simulink model "BEV_maxSpeed"  (R2023a)
settings: Solver=FixedStepAuto  StartTime=0.0  StopTime=1000  FixedStep=1  RelTol=1e-3
undefined symbols (not defined in the file): acceleration_threshold, attributes, battery_GD, config_gearbox, config_Inverter, config_motor, config_vehicle, efficiency_vector, efficiency_vector2, GB, gearbox_map, k_FW, lossData, lossData2, max_torque_map, max_torque_map2, speed_vector, speed_vector2
libraries: spsParallelRLCBranchLib x20, spsControlledCurrentSourceLib x8, spsVoltageMeasurementLib x8, simulink x4, spsDCVoltageSourceLib x4, spspowerguiLib x4, eePmsmCurrentReferenceGen x2
(part 1 of 2)
settings Model: PauseTimes=35  Creator=maximilian.tschochne  LastModifiedBy=polashehata
settings OptimizationCC: ReuseModelBlockBuffer=off
settings DebuggingCC: MergeDetectMultiDrivingBlocksExec=none
settings ModelReferenceCC: PropagateSignalLabelsOutOfModel=off
settings RTWCC: GenCodeOnly=on  GenerateReport=on  BuildConfiguration=Faster Runs  CheckMdlBeforeBuild=Warning
settings GRTTargetCC: TargetLangStandard=C89/C90 (ANSI)  CodeInterfacePackaging=Reusable function  GenerateAllocFcn=on

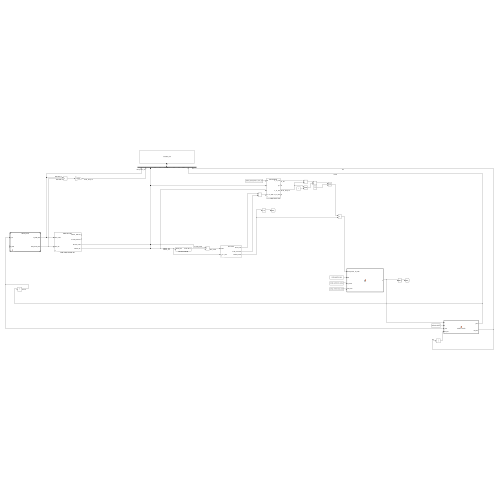
[thumbnail: Simulink's stored preview of the top-level diagram]
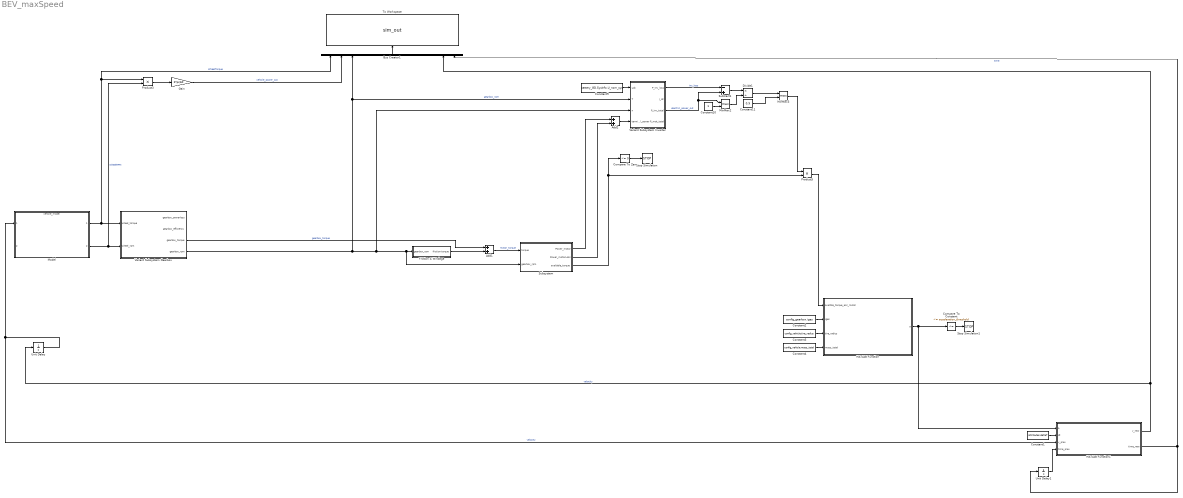
== system BEV_maxSpeed ==
  Add1 : Sum
  Add2 : Sum
  Bus Creator1 : BusCreator  Inputs=12
  Compare To Constant : simulink/Logic and Bit Operations/Compare To Constant  relop=<=  const=acceleration_threshold  OutDataTypeStr=boolean
  Compare To Zero : simulink/Logic and Bit Operations/Compare To Zero  relop=<=  OutDataTypeStr=boolean
  Constant1 : Constant  Value=attributes.deltaT
  Constant10 : Constant
  Constant11 : Constant  Value=0.9
  Constant2 : Constant  Value=config_gearbox.iges
  Constant3 : Constant  Value=config_vehicle.tire_radius
  Constant4 : Constant  Value=config_vehicle.mass_total
  Constant9 : Constant  Value=battery_GD.SysInfo.U_nom_sys
  Divide1 : Product  Inputs=*/
  Friction & Windage : Subsystem
  Gain : Gain  Gain=2*pi/60
  MATLAB Function : MATLAB Function  TreatAsAtomicUnit=on
  MATLAB Function1 : MATLAB Function  TreatAsAtomicUnit=on
  MinMax2 : MinMax  Function=max  Inputs=2
  MinMax3 : MinMax  Function=max  Inputs=2
  Model : ModelReference  ModelNameDialog=vehicle_model.slx  SimulationMode=Normal  ModelReferenceVersion=4.1
  Product3 : Product
  Product5 : Product
  Stop Simulation : Stop
  Stop Simulation1 : Stop
  Subsystem : Subsystem  Variant=on  VariantControl=Subsystem
  Subtract1 : Sum  Inputs=-+
  To Workspace : ToWorkspace  VariableName=sim_out  SaveFormat=Timeseries  SampleTime=-1
  Unit Delay : UnitDelay  SampleTime=-1  HasFrameUpgradeWarning=on
  Unit Delay1 : UnitDelay  SampleTime=-1  HasFrameUpgradeWarning=on
  Variant Subsystem Gearbox : Subsystem  Variant=on
  Variant Subsystem Inverter : Subsystem  Variant=on
  wires:
  Bus Creator1/1 -> To Workspace/1
  Gain/1 -> Bus Creator1/2  "vehicle_power_out"
  Model/2 -> Product3/2, Variant Subsystem Gearbox/2(wheel_rpm)  "WheelRPM"
  Model/1 -> Bus Creator1/1, Product3/1, Variant Subsystem Gearbox/1(wheel_torque)  "WheelTorque"
  Product3/1 -> Gain/1
  Constant1/1 -> MATLAB Function1/2(dt)
  MATLAB Function/1(a) -> MATLAB Function1/1(a), Compare To Constant/1
  MATLAB Function1/1(v_new) -> Unit Delay/1, Bus Creator1/11  "velocity"
  MATLAB Function1/2(time_new) -> Bus Creator1/12, Unit Delay1/1  "time"
  Add1/1 -> Subsystem/1(torque)  "motor_torque"
  Variant Subsystem Gearbox/3(gearbox_torque) -> Add1/1  "gearbox_torque"
  Variant Subsystem Gearbox/4(gearbox_rpm) -> Subsystem/2(gearbox_rpm), Friction & Windage/1(gearbox_rpm), Variant Subsystem Inverter/3(n), Bus Creator1/3, Variant Subsystem Inverter/2(T)  "gearbox_rpm"
  Friction & Windage/1(friction torque) -> Add1/2
  Constant2/1 -> MATLAB Function/2(iges)
  Constant3/1 -> MATLAB Function/3(tire_radius)
  Constant4/1 -> MATLAB Function/4(mass_total)
  Unit Delay1/1 -> MATLAB Function1/4(time_prev)
  Unit Delay/1 -> Model/1, MATLAB Function1/3(v_prev)  "velocity"
  Compare To Zero/1 -> Stop Simulation/1
  Compare To Constant/1 -> Stop Simulation1/1
  Constant9/1 -> Variant Subsystem Inverter/1(udc)
  Add2/1 -> Variant Subsystem Inverter/4(terminal_power)
  Variant Subsystem Inverter/3(P_inv_total) -> Subtract1/2, MinMax2/1  "electric_power_out"
  Variant Subsystem Inverter/1(P_inv_loss) -> Subtract1/1  "inv_loss"
  Subtract1/1 -> Divide1/1
  Divide1/1 -> MinMax3/1
  Product5/1 -> MATLAB Function/1(availble_torque_acc_motor)
  Constant10/1 -> MinMax2/2
  MinMax2/1 -> Divide1/2
  Constant11/1 -> MinMax3/2
  MinMax3/1 -> Product5/1
  Subsystem/1(Power_motor) -> Add2/1
  Subsystem/2(Power_motorLoss) -> Add2/2
  Subsystem/3(available_torque) -> Product5/2, Compare To Zero/1

== system BEV_maxSpeed/Friction & Windage ==
  note: Gleichung für mechanische Verlustleistung:
      | P_FW = k_FW * n^2.5
  gearbox_rpm : Inport
  Constant : Constant  Value=2.5
  Constant1 : Constant  Value=0
  Constant5 : Constant  Value=k_FW
  Gain : Gain  Gain=2*pi/60
  In2 : InportShadow
  Power : Math  Operator=pow
  Product : Product
  Product2 : Product  Inputs=*/
  Switch : Switch  Criteria=u2 > Threshold  SaturateOnIntegerOverflow=off  InputSameDT=off
  friction torque : Outport
  wires:
  gearbox_rpm/1 -> Power/1  "n_gearbox"
  Constant/1 -> Power/2  "exponent"
  Power/1 -> Product/1
  Constant5/1 -> Product/2
  Product/1 -> Product2/1  "mech powerloss"
  Product2/1 -> Switch/1  "torque"
  In2/1 -> Gain/1  "n_gearbox"
  Gain/1 -> Product2/2, Switch/2
  Switch/1 -> friction torque/1
  Constant1/1 -> Switch/3

== system BEV_maxSpeed/Subsystem ==
  torque : Inport
  gearbox_rpm : Inport  Port=2
  One Motor : Subsystem  VariantControl="Motor_Mode == \"LookupOneMotor\""
  Two motors : Subsystem  VariantControl="Motor_Mode == \"Lookup\""
  Power_motor : Outport
  Power_motorLoss : Outport  Port=2
  available_torque : Outport  Port=3

== system BEV_maxSpeed/Variant Subsystem Gearbox ==
  note: 1) Add Subsystem or Model blocks as valid variant choices.
      | 2) You cannot connect blocks at this level. At simulation, connectivity is automatically
      | determined, based on the active variant and port name matching.
  wheel_torque : Inport
  wheel_rpm : Inport  Port=2
  Gearbox Analytic : Subsystem  VariantControl="GB_Mode == \"Analytic\""
  Gearbox Const : Subsystem  VariantControl="GB_Mode == \"Const\""
  Gearbox Lookup-Table : Subsystem  VariantControl="GB_Mode == \"Lookup\""
  Gearbox Simple : Subsystem  VariantControl="GB_Mode == \"Simple\""
  gearbox_powerloss : Outport
  gearbox_efficiency : Outport  Port=2
  gearbox_torque : Outport  Port=3
  gearbox_rpm : Outport  Port=4

== system BEV_maxSpeed/Variant Subsystem Inverter ==
  note: 1) Add Subsystem or Model blocks as valid variant choices.
      | 2) You cannot connect blocks at this level. At simulation, connectivity is automatically
      | determined, based on the active variant and port name matching.
  udc : Inport
  T : Inport  Port=2
  n : Inport  Port=3
  terminal_power : Inport  Port=4
  Inverter Analytic : Subsystem  VariantControl="Inverter_Mode == \"Analytic\""
  Inverter Simple : Subsystem  VariantControl="Inverter_Mode == \"Simple\""
  P_inv_loss : Outport
  I_dc : Outport  Port=2
  P_inv_total : Outport  Port=3
  P_mot_total : Outport  Port=4

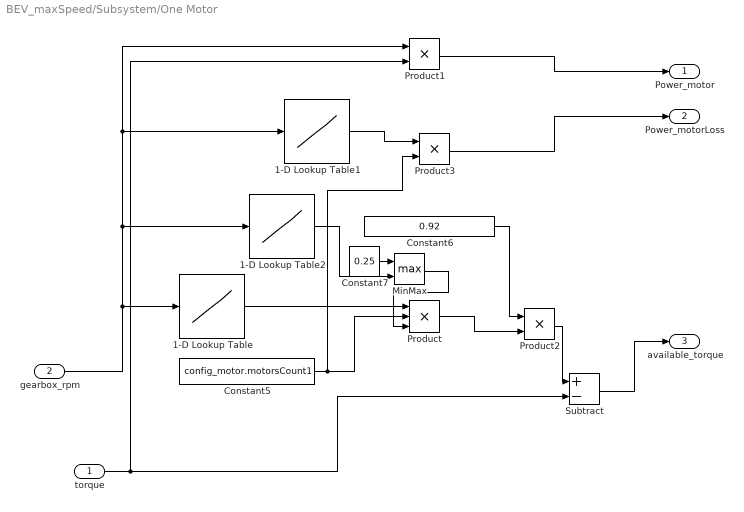
== system BEV_maxSpeed/Subsystem/One Motor ==
  torque : Inport
  gearbox_rpm : Inport  Port=2
  1-D Lookup Table : Lookup_n-D  NumberOfTableDimensions=1  BreakpointsForDimension1=speed_vector  Table=max_torque_map  InternalRulePriority=Speed  RndMeth=Simplest
  1-D Lookup Table1 : Lookup_n-D  NumberOfTableDimensions=1  BreakpointsForDimension1=speed_vector  Table=lossData  InternalRulePriority=Speed  RndMeth=Simplest
  1-D Lookup Table2 : Lookup_n-D  NumberOfTableDimensions=1  BreakpointsForDimension1=speed_vector  Table=efficiency_vector  InternalRulePriority=Speed  RndMeth=Simplest
  Constant5 : Constant  Value=config_motor.motorsCount1
  Constant6 : Constant  Value=0.92
  Constant7 : Constant  Value=0.25
  MinMax : MinMax  Function=max  Inputs=2
  Product : Product  Inputs=3
  Product1 : Product
  Product2 : Product
  Product3 : Product
  Subtract : Sum  Inputs=+-
  Power_motor : Outport
  Power_motorLoss : Outport  Port=2
  available_torque : Outport  Port=3
  wires:
  Product2/1 -> Subtract/1
  Subtract/1 -> available_torque/1
  1-D Lookup Table2/1 -> MinMax/2
  Constant5/1 -> Product/2, Product3/2
  Constant7/1 -> MinMax/1
  MinMax/1 -> Product/3
  1-D Lookup Table/1 -> Product/1
  Constant6/1 -> Product2/1
  Product/1 -> Product2/2
  gearbox_rpm/1 -> 1-D Lookup Table/1, 1-D Lookup Table2/1, Product1/1, 1-D Lookup Table1/1
  torque/1 -> Product1/2, Subtract/2
  1-D Lookup Table1/1 -> Product3/1
  Product3/1 -> Power_motorLoss/1
  Product1/1 -> Power_motor/1

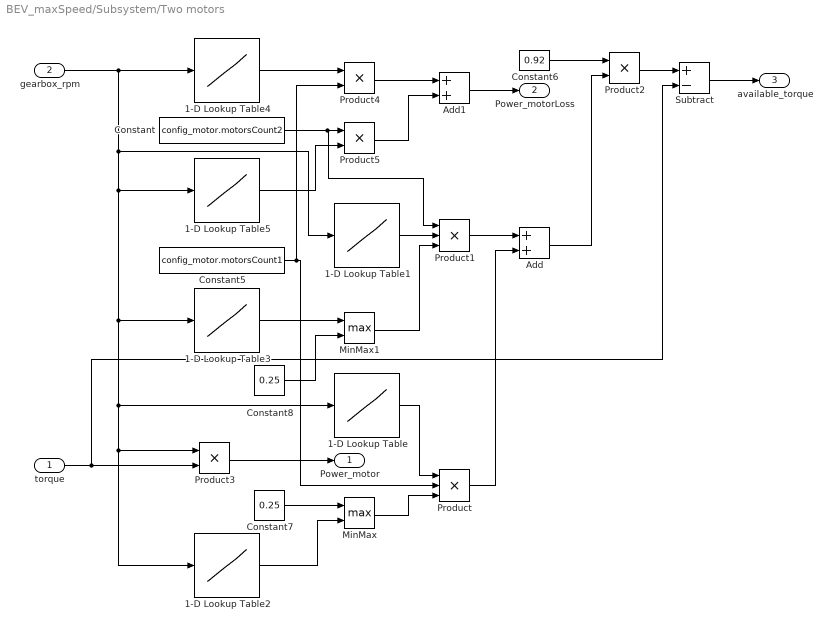
== system BEV_maxSpeed/Subsystem/Two motors ==
  torque : Inport
  gearbox_rpm : Inport  Port=2
  1-D Lookup Table : Lookup_n-D  NumberOfTableDimensions=1  BreakpointsForDimension1=speed_vector  Table=max_torque_map  InternalRulePriority=Speed  RndMeth=Simplest
  1-D Lookup Table1 : Lookup_n-D  NumberOfTableDimensions=1  BreakpointsForDimension1=speed_vector2  Table=max_torque_map2  InternalRulePriority=Speed  RndMeth=Simplest
  1-D Lookup Table2 : Lookup_n-D  NumberOfTableDimensions=1  BreakpointsForDimension1=speed_vector  Table=efficiency_vector  InternalRulePriority=Speed  RndMeth=Simplest
  1-D Lookup Table3 : Lookup_n-D  NumberOfTableDimensions=1  BreakpointsForDimension1=speed_vector2  Table=efficiency_vector2  InternalRulePriority=Speed  RndMeth=Simplest
  1-D Lookup Table4 : Lookup_n-D  NumberOfTableDimensions=1  BreakpointsForDimension1=speed_vector  Table=lossData  InternalRulePriority=Speed  RndMeth=Simplest
  1-D Lookup Table5 : Lookup_n-D  NumberOfTableDimensions=1  BreakpointsForDimension1=speed_vector2  Table=lossData2  InternalRulePriority=Speed  RndMeth=Simplest
  Add : Sum
  Add1 : Sum
  Constant : Constant  Value=config_motor.motorsCount2
  Constant5 : Constant  Value=config_motor.motorsCount1
  Constant6 : Constant  Value=0.92
  Constant7 : Constant  Value=0.25
  Constant8 : Constant  Value=0.25
  MinMax : MinMax  Function=max  Inputs=2
  MinMax1 : MinMax  Function=max  Inputs=2
  Product : Product  Inputs=3
  Product1 : Product  Inputs=3
  Product{2..5} (4 alike) : Product
  Subtract : Sum  Inputs=+-
  Power_motor : Outport
  Power_motorLoss : Outport  Port=2
  available_torque : Outport  Port=3
  wires:
  Subtract/1 -> available_torque/1
  1-D Lookup Table2/1 -> MinMax/2
  Product2/1 -> Subtract/1
  Add/1 -> Product2/2
  Constant6/1 -> Product2/1
  Product/1 -> Add/2
  Add1/1 -> Power_motorLoss/1
  1-D Lookup Table1/1 -> Product1/2
  Product5/1 -> Add1/2
  Constant7/1 -> MinMax/1
  MinMax/1 -> Product/3
  Product3/1 -> Power_motor/1
  Constant8/1 -> MinMax1/2
  1-D Lookup Table3/1 -> MinMax1/1
  Product1/1 -> Add/1
  Constant5/1 -> Product4/2, Product/2
  1-D Lookup Table4/1 -> Product4/1
  1-D Lookup Table/1 -> Product/1
  Constant/1 -> Product5/1, Product1/1
  torque/1 -> Product3/2, Subtract/2
  MinMax1/1 -> Product1/3
  Product4/1 -> Add1/1
  1-D Lookup Table5/1 -> Product5/2
  gearbox_rpm/1 -> Product3/1, 1-D Lookup Table2/1, 1-D Lookup Table/1, 1-D Lookup Table3/1, 1-D Lookup Table5/1, 1-D Lookup Table1/1, 1-D Lookup Table4/1

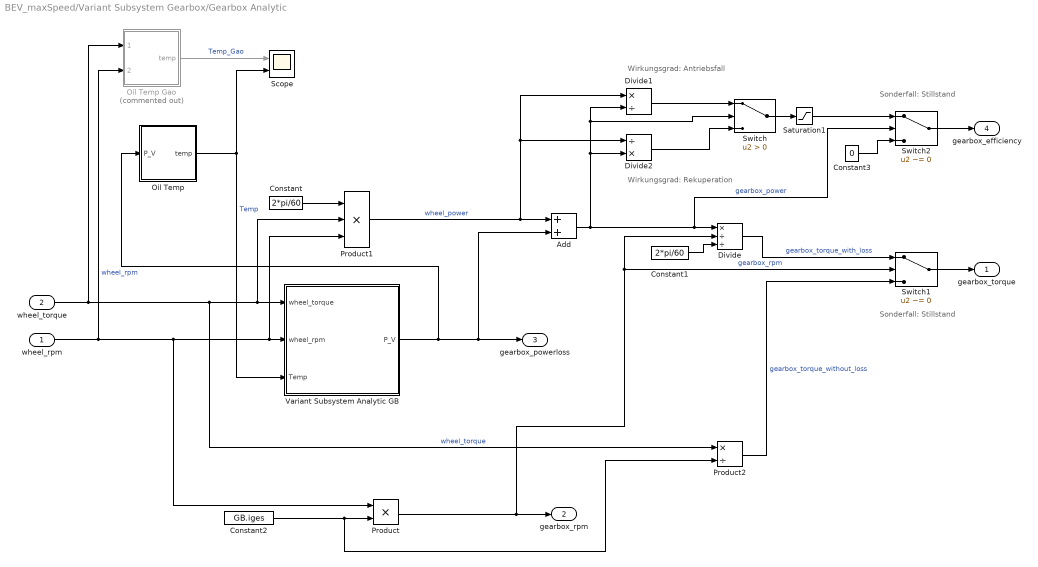
== system BEV_maxSpeed/Variant Subsystem Gearbox/Gearbox Analytic ==
  note: Wirkungsgrad:
      | Antriebsfall
  note: Sonderfall: Stillstand
  note: Sonderfall: Stillstand
  note: Wirkungsgrad:
      | Rekuperation
  wheel_rpm : Inport
  wheel_torque : Inport  Port=2
  Add : Sum
  Constant : Constant  Value=2*pi/60
  Constant1 : Constant  Value=2*pi/60
  Constant2 : Constant  Value=GB.iges
  Constant3 : Constant  Value=0
  Divide : Product  Inputs=*//
  Divide1 : Product  Inputs=*/
  Divide2 : Product  Inputs=/*
  Oil Temp : Subsystem
  Oil Temp Gao : Subsystem  Commented=on
  Product : Product
  Product1 : Product  Inputs=3
  Product2 : Product  Inputs=*/
  Saturation1 : Saturate  UpperLimit=inf  LowerLimit=0
  Scope : Scope  NumInputPorts=2
  Switch : Switch  Criteria=u2 > Threshold  SaturateOnIntegerOverflow=off  InputSameDT=off
  Switch1 : Switch  Criteria=u2 ~= 0  SaturateOnIntegerOverflow=off  InputSameDT=off
  Switch2 : Switch  Criteria=u2 ~= 0  SaturateOnIntegerOverflow=off  InputSameDT=off
  Variant Subsystem Analytic GB : Subsystem  Variant=on
  gearbox_torque : Outport
  gearbox_rpm : Outport  Port=2
  gearbox_powerloss : Outport  Port=3
  gearbox_efficiency : Outport  Port=4
  wires:
  wheel_torque/1 -> Variant Subsystem Analytic GB/1(wheel_torque), Product1/2, Product2/1, Oil Temp Gao/1(T_wheel)  "wheel_torque"
  wheel_rpm/1 -> Product/1, Variant Subsystem Analytic GB/2(wheel_rpm), Product1/3, Oil Temp Gao/2(rpm_wheel)  "wheel_rpm"
  Variant Subsystem Analytic GB/1(P_V) -> Oil Temp/1(P_V), Add/2, gearbox_powerloss/1
  Constant2/1 -> Product2/2, Product/2
  Product/1 -> Switch1/2, Divide/2, gearbox_rpm/1  "gearbox_rpm"
  Constant/1 -> Product1/1
  Product1/1 -> Divide2/1, Divide1/1, Add/1  "wheel_power"
  Add/1 -> Divide2/2, Switch/2, Divide1/2, Switch2/2, Divide/1  "gearbox_power"
  Constant1/1 -> Divide/3
  Divide/1 -> Switch1/1  "gearbox_torque_with_loss"
  Switch/1 -> Saturation1/1
  Divide2/1 -> Switch/3
  Switch1/1 -> gearbox_torque/1
  Product2/1 -> Switch1/3  "gearbox_torque_without_loss"
  Switch2/1 -> gearbox_efficiency/1
  Constant3/1 -> Switch2/3
  Divide1/1 -> Switch/1
  Oil Temp Gao/1(temp) -> Scope/1  "Temp_Gao"
  Oil Temp/1(temp) -> Scope/2, Variant Subsystem Analytic GB/3(Temp)  "Temp"
  Saturation1/1 -> Switch2/1

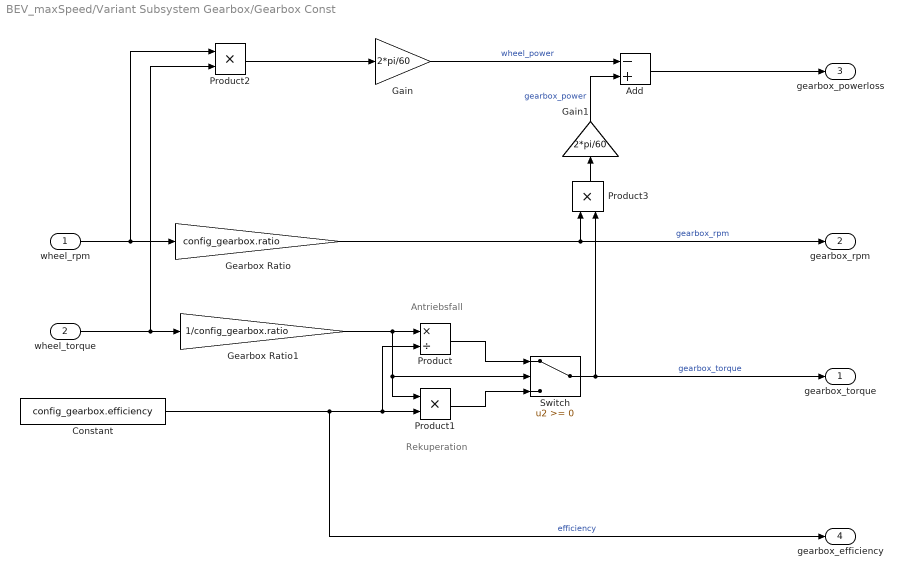
== system BEV_maxSpeed/Variant Subsystem Gearbox/Gearbox Const ==
  note: Rekuperation
  note: Antriebsfall
  wheel_rpm : Inport
  wheel_torque : Inport  Port=2
  Add : Sum  Inputs=-+
  Constant : Constant  Value=config_gearbox.efficiency
  Gain : Gain  Gain=2*pi/60
  Gain1 : Gain  Gain=2*pi/60
  Gearbox Ratio : Gain  Gain=config_gearbox.ratio
  Gearbox Ratio1 : Gain  Gain=1/config_gearbox.ratio
  Product : Product  Inputs=*/
  Product1 : Product  Inputs=**
  Product2 : Product
  Product3 : Product
  Switch : Switch  SaturateOnIntegerOverflow=off  InputSameDT=off
  gearbox_torque : Outport
  gearbox_rpm : Outport  Port=2
  gearbox_powerloss : Outport  Port=3
  gearbox_efficiency : Outport  Port=4
  wires:
  wheel_rpm/1 -> Product2/1, Gearbox Ratio/1
  Gearbox Ratio/1 -> gearbox_rpm/1, Product3/1  "gearbox_rpm"
  wheel_torque/1 -> Product2/2, Gearbox Ratio1/1
  Gearbox Ratio1/1 -> Product1/1, Switch/2, Product/1
  Constant/1 -> gearbox_efficiency/1, Product1/2, Product/2  "efficiency"
  Product/1 -> Switch/1
  Product1/1 -> Switch/3
  Switch/1 -> gearbox_torque/1, Product3/2  "gearbox_torque"
  Product2/1 -> Gain/1
  Add/1 -> gearbox_powerloss/1
  Product3/1 -> Gain1/1
  Gain/1 -> Add/1  "wheel_power"
  Gain1/1 -> Add/2  "gearbox_power"

== system BEV_maxSpeed/Variant Subsystem Gearbox/Gearbox Lookup-Table ==
  wheel_rpm : Inport
  wheel_torque : Inport  Port=2
  Oil Temp : Subsystem
  Oil Temp Gao : Subsystem  Commented=on
  Scope : Scope  Commented=on  NumInputPorts=2
  Variant Subsystem : Subsystem  Variant=on
  gearbox_torque : Outport
  gearbox_rpm : Outport  Port=2
  gearbox_powerloss : Outport  Port=3
  gearbox_efficiency : Outport  Port=4
  wires:
  Oil Temp Gao/1(temp) -> Scope/2
  wheel_torque/1 -> Oil Temp Gao/1(T_wheel), Variant Subsystem/1(wheel_torque)  "wheel_torque"
  wheel_rpm/1 -> Oil Temp Gao/2(rpm_wheel), Variant Subsystem/2(wheel_rpm)  "wheel_rpm"
  Variant Subsystem/4(gearbox_torque) -> gearbox_torque/1
  Variant Subsystem/1(loss_lockup) -> Oil Temp/1(P_V), gearbox_powerloss/1
  Variant Subsystem/3(gearbox_rpm) -> gearbox_rpm/1
  Variant Subsystem/2(gearbox_efficiency) -> gearbox_efficiency/1
  Oil Temp/1(temp) -> Scope/1, Variant Subsystem/3(Temp)

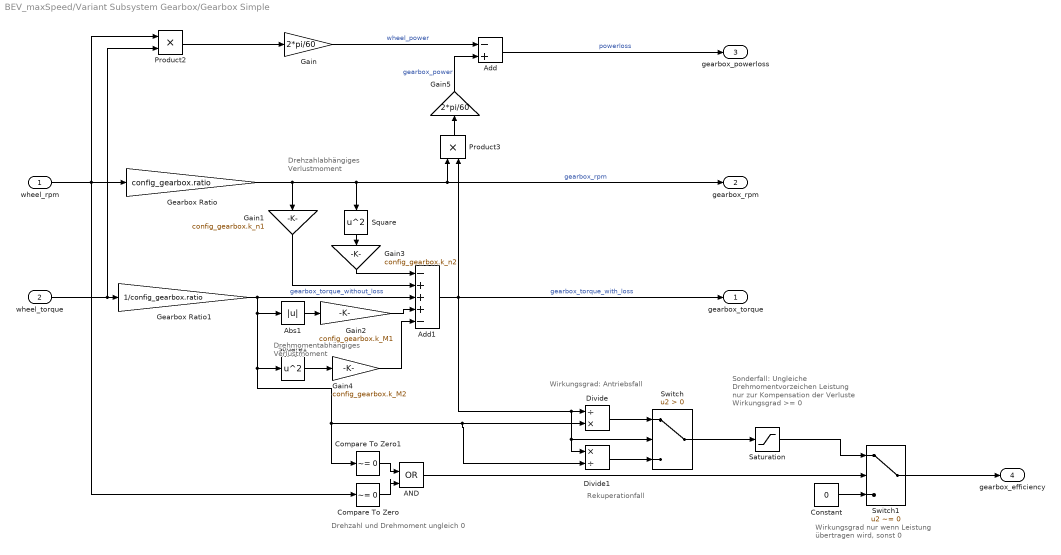
== system BEV_maxSpeed/Variant Subsystem Gearbox/Gearbox Simple ==
  note: Rekuperationfall
  note: Sonderfall: Ungleiche Drehmomentvorzeichen
      | Leistung nur zur Kompensation der Verluste
      | Wirkungsgrad >= 0
  note: Drehzahl und Drehmoment ungleich 0
  note: Drehmomentabhängiges
      | Verlustmoment
  note: Drehzahlabhängiges
      | Verlustmoment
  note: Wirkungsgrad nur wenn Leistung
      | übertragen wird, sonst 0
  note: Wirkungsgrad: Antriebsfall
  wheel_rpm : Inport
  wheel_torque : Inport  Port=2
  AND : Logic  Operator=OR  IconShape=distinctive  AllPortsSameDT=off  OutDataTypeStr=boolean
  Abs1 : Abs  SaturateOnIntegerOverflow=off
  Add : Sum  Inputs=-+
  Add1 : Sum  Inputs=-+++-
  Compare To Zero : simulink/Logic and Bit Operations/Compare To Zero  relop=~=  OutDataTypeStr=boolean
  Compare To Zero1 : simulink/Logic and Bit Operations/Compare To Zero  relop=~=  OutDataTypeStr=boolean
  Constant : Constant  Value=0
  Divide : Product  Inputs=/*
  Divide1 : Product  Inputs=*/
  Gain : Gain  Gain=2*pi/60
  Gain1 : Gain  Gain=config_gearbox.k_n1
  Gain2 : Gain  Gain=config_gearbox.k_M1
  Gain3 : Gain  Gain=config_gearbox.k_n2
  Gain4 : Gain  Gain=config_gearbox.k_M2
  Gain5 : Gain  Gain=2*pi/60
  Gearbox Ratio : Gain  Gain=config_gearbox.ratio
  Gearbox Ratio1 : Gain  Gain=1/config_gearbox.ratio
  Product2 : Product
  Product3 : Product
  Saturation : Saturate  UpperLimit=inf  LowerLimit=0
  Square : Math  Operator=square
  Square1 : Math  Operator=square
  Switch : Switch  Criteria=u2 > Threshold  SaturateOnIntegerOverflow=off  InputSameDT=off
  Switch1 : Switch  Criteria=u2 ~= 0  SaturateOnIntegerOverflow=off  InputSameDT=off
  gearbox_torque : Outport
  gearbox_rpm : Outport  Port=2
  gearbox_powerloss : Outport  Port=3
  gearbox_efficiency : Outport  Port=4
  wires:
  Product3/1 -> Gain5/1
  Add/1 -> gearbox_powerloss/1  "powerloss"
  Add1/1 -> Product3/2, gearbox_torque/1, Switch/2, Divide1/1, Divide/1  "gearbox_torque_with_loss"
  wheel_torque/1 -> Product2/2, Gearbox Ratio1/1
  Gearbox Ratio/1 -> Square/1, Product3/1, gearbox_rpm/1, Gain1/1  "gearbox_rpm"
  wheel_rpm/1 -> Compare To Zero/1, Gearbox Ratio/1, Product2/1
  Gearbox Ratio1/1 -> Abs1/1, Square1/1, Compare To Zero1/1, Divide1/2, Divide/2, Add1/3  "gearbox_torque_without_loss"
  Gain1/1 -> Add1/2
  Gain2/1 -> Add1/4
  Abs1/1 -> Gain2/1
  Divide/1 -> Switch/1
  Switch/1 -> Saturation/1
  Divide1/1 -> Switch/3
  Constant/1 -> Switch1/3
  Gain3/1 -> Add1/1
  Square/1 -> Gain3/1
  Switch1/1 -> gearbox_efficiency/1
  Square1/1 -> Gain4/1
  Gain4/1 -> Add1/5
  Compare To Zero1/1 -> AND/1
  Compare To Zero/1 -> AND/2
  AND/1 -> Switch1/2
  Product2/1 -> Gain/1
  Gain/1 -> Add/1  "wheel_power"
  Gain5/1 -> Add/2  "gearbox_power"
  Saturation/1 -> Switch1/1

== system BEV_maxSpeed/Variant Subsystem Inverter/Inverter Analytic ==
  udc : Inport
  T : Inport  Port=2
  n : Inport  Port=3
  terminal_power : Inport  Port=4
  Variant Subsystem : Subsystem  Variant=on
  P_inv_loss : Outport
  I_dc : Outport  Port=2
  P_inv_total : Outport  Port=3
  P_mot_total : Outport  Port=4
  wires:
  Variant Subsystem/4(P_mot_elec) -> P_mot_total/1
  Variant Subsystem/3(P_inv_total) -> P_inv_total/1
  Variant Subsystem/2(idc) -> I_dc/1
  Variant Subsystem/1(Conduction_and_Switching_loss) -> P_inv_loss/1
  T/1 -> Variant Subsystem/3(torque)
  n/1 -> Variant Subsystem/2(rpm)
  udc/1 -> Variant Subsystem/1(udc)
  terminal_power/1 -> Variant Subsystem/4(terminal_power)

== system BEV_maxSpeed/Variant Subsystem Inverter/Inverter Simple ==
  T : Inport
  n : Inport  Port=2
  udc : Inport  Port=3
  terminal_power : Inport  Port=4
  MATLAB Function : MATLAB Function  TreatAsAtomicUnit=on
  P_inv_loss : Outport
  I_dc : Outport  Port=2
  P_inv_total : Outport  Port=3
  P_mot_total : Outport  Port=4
  wires:
  T/1 -> MATLAB Function/1(T)
  n/1 -> MATLAB Function/2(n)
  udc/1 -> MATLAB Function/3(udc)
  terminal_power/1 -> MATLAB Function/4(P_Terminal)
  MATLAB Function/1(P_inv_loss) -> P_inv_loss/1
  MATLAB Function/2(I_dc) -> I_dc/1
  MATLAB Function/3(P_inv_total) -> P_inv_total/1
  MATLAB Function/4(P_mot_total) -> P_mot_total/1

== system BEV_maxSpeed/Variant Subsystem Gearbox/Gearbox Analytic/Oil Temp ==
  P_V : Inport
  IC : InitialCondition  Value=25
  MATLAB Function : MATLAB Function  TreatAsAtomicUnit=on
  Memory1 : Memory  InitialCondition=config_vehicle.ambient_temp - 273
  Memory2 : Memory  InitialCondition=config_vehicle.ambient_temp - 273
  Scope : Scope
  temp : Outport
  wires:
  MATLAB Function/1(T) -> IC/1  "GB_temp"
  Memory1/1 -> MATLAB Function/1(t)
  P_V/1 -> Memory2/1
  IC/1 -> Scope/1, Memory1/1, temp/1
  Memory2/1 -> MATLAB Function/2(P_V)

== system BEV_maxSpeed/Variant Subsystem Gearbox/Gearbox Analytic/Oil Temp Gao ==
  note: entspricht 2pi/60 * 1e-3
  T_wheel : Inport
  rpm_wheel : Inport  Port=2
  MATLAB Function : MATLAB Function  TreatAsAtomicUnit=on
  Memory1 : Memory  InitialCondition=config_vehicle.ambient_temp - 273
  Multiply5 : Gain  Gain=1/9550
  Product2 : Product
  Scope : Scope
  temp : Outport
  wires:
  Product2/1 -> Multiply5/1
  rpm_wheel/1 -> MATLAB Function/3(rpm), Product2/2
  T_wheel/1 -> Product2/1
  MATLAB Function/1(T) -> Scope/1, Memory1/1, temp/1
  Memory1/1 -> MATLAB Function/1(t)
  Multiply5/1 -> MATLAB Function/2(P)

== system BEV_maxSpeed/Variant Subsystem Gearbox/Gearbox Analytic/Variant Subsystem Analytic GB ==
  note: 1) Add Subsystem or Model blocks as valid variant choices.
      | 2) You cannot connect blocks at this level. At simulation, connectivity is automatically
      | determined, based on the active variant and port name matching.
  wheel_torque : Inport
  wheel_rpm : Inport  Port=2
  Temp : Inport  Port=3
  Einstufig_Achsparallel : Subsystem  VariantControl=GB_Stufen == 1
  Zweistufig_Achsparallel : Subsystem  VariantControl="GB_Stufen == 2 && GB_Topology == \"achsparallel\""
  Zweistufig_Koaxial : Subsystem  VariantControl="GB_Stufen == 2 && GB_Topology == \"koaxial\""
  P_V : Outport

== system BEV_maxSpeed/Variant Subsystem Gearbox/Gearbox Lookup-Table/Oil Temp ==
  P_V : Inport
  IC : InitialCondition  Value=25
  MATLAB Function : MATLAB Function  TreatAsAtomicUnit=on
  Memory1 : Memory  InitialCondition=config_vehicle.ambient_temp - 273
  Memory2 : Memory  InitialCondition=config_vehicle.ambient_temp - 273
  Scope : Scope
  temp : Outport
  wires:
  MATLAB Function/1(T) -> IC/1  "GB_temp"
  Memory1/1 -> MATLAB Function/1(t)
  P_V/1 -> Memory2/1
  IC/1 -> Scope/1, Memory1/1, temp/1
  Memory2/1 -> MATLAB Function/2(P_V)

== system BEV_maxSpeed/Variant Subsystem Gearbox/Gearbox Lookup-Table/Oil Temp Gao ==
  note: entspricht 2pi/60 * 1e-3
  T_wheel : Inport
  rpm_wheel : Inport  Port=2
  MATLAB Function : MATLAB Function  TreatAsAtomicUnit=on
  Memory1 : Memory  InitialCondition=config_vehicle.ambient_temp - 273
  Multiply5 : Gain  Gain=1/9550
  Product2 : Product
  Scope : Scope
  temp : Outport
  wires:
  Product2/1 -> Multiply5/1
  rpm_wheel/1 -> MATLAB Function/3(rpm), Product2/2
  T_wheel/1 -> Product2/1
  MATLAB Function/1(T) -> Scope/1, Memory1/1, temp/1
  Memory1/1 -> MATLAB Function/1(t)
  Multiply5/1 -> MATLAB Function/2(P)

== system BEV_maxSpeed/Variant Subsystem Gearbox/Gearbox Lookup-Table/Variant Subsystem ==
  note: 1) Add Subsystem or Model blocks as valid variant choices.
      | 2) You cannot connect blocks at this level. At simulation, connectivity is automatically
      | determined, based on the active variant and port name matching.
  wheel_torque : Inport
  wheel_rpm : Inport  Port=2
  Temp : Inport  Port=3
  ETA_map : Subsystem  VariantControl="gearbox_map.map_type == \"Eta\""
  LOSS_map : Subsystem  VariantControl="gearbox_map.map_type == \"Loss\""
  loss_lockup : Outport
  gearbox_efficiency : Outport  Port=2
  gearbox_rpm : Outport  Port=3
  gearbox_torque : Outport  Port=4

== system BEV_maxSpeed/Variant Subsystem Inverter/Inverter Analytic/Variant Subsystem ==
  note: 1) Add Subsystem or Model blocks as valid variant choices.
      | 2) You cannot connect blocks at this level. At simulation, connectivity is automatically
      | determined, based on the active variant and port name matching.
  udc : Inport
  rpm : Inport  Port=2
  torque : Inport  Port=3
  terminal_power : Inport  Port=4
  IM_Inverter_IGBT_Analytic : Subsystem  VariantControl=Mode_IM_IGBT
  IM_Inverter_SiC-MOSFET_Analytic : Subsystem  VariantControl=Mode_IM_MOSFET
  PMSM_Inverter_IBGT_Analytic : Subsystem  VariantControl=Mode_PSM_IGBT
  PMSM_Inverter_SiC-MOSFET_Analytic : Subsystem  VariantControl=Mode_PSM_MOSFET
  Conduction_and_Switching_loss : Outport
  idc : Outport  Port=2
  P_inv_total : Outport  Port=3
  P_mot_elec : Outport  Port=4

== system BEV_maxSpeed/Variant Subsystem Gearbox/Gearbox Analytic/Variant Subsystem Analytic GB/Einstufig_Achsparallel ==
  wheel_torque : Inport
  wheel_rpm : Inport  Port=2
  Temp : Inport  Port=3
  Add : Sum
  MATLAB Function : MATLAB Function  TreatAsAtomicUnit=on
  Ölpumpe : Subsystem
  P_V : Outport
  wires:
  wheel_rpm/1 -> Ölpumpe/1(nrad), MATLAB Function/2(nrad)
  MATLAB Function/1(P_V) -> Add/1
  wheel_torque/1 -> MATLAB Function/1(Mrad)
  Temp/1 -> MATLAB Function/3(Temp)
  Add/1 -> P_V/1
  Ölpumpe/1(power_oilpump) -> Add/2

== system BEV_maxSpeed/Variant Subsystem Gearbox/Gearbox Analytic/Variant Subsystem Analytic GB/Zweistufig_Achsparallel ==
  wheel_torque : Inport
  wheel_rpm : Inport  Port=2
  Temp : Inport  Port=3
  Add : Sum
  MATLAB Function : MATLAB Function  TreatAsAtomicUnit=on
  Ölpumpe : Subsystem
  P_V : Outport
  wires:
  wheel_rpm/1 -> Ölpumpe/1(nrad), MATLAB Function/2(nrad)
  MATLAB Function/1(P_V) -> Add/1
  wheel_torque/1 -> MATLAB Function/1(Mrad)
  Temp/1 -> MATLAB Function/3(Temp)
  Add/1 -> P_V/1
  Ölpumpe/1(power_oilpump) -> Add/2

== system BEV_maxSpeed/Variant Subsystem Gearbox/Gearbox Analytic/Variant Subsystem Analytic GB/Zweistufig_Koaxial ==
  wheel_torque : Inport
  wheel_rpm : Inport  Port=2
  Temp : Inport  Port=3
  Add : Sum
  MATLAB Function : MATLAB Function  TreatAsAtomicUnit=on
  Ölpumpe : Subsystem
  P_V : Outport
  wires:
  Temp/1 -> MATLAB Function/3(Temp)
  wheel_torque/1 -> MATLAB Function/1(Mrad)
  MATLAB Function/1(P_V) -> Add/1
  wheel_rpm/1 -> Ölpumpe/1(nrad), MATLAB Function/2(nrad)
  Add/1 -> P_V/1
  Ölpumpe/1(power_oilpump) -> Add/2

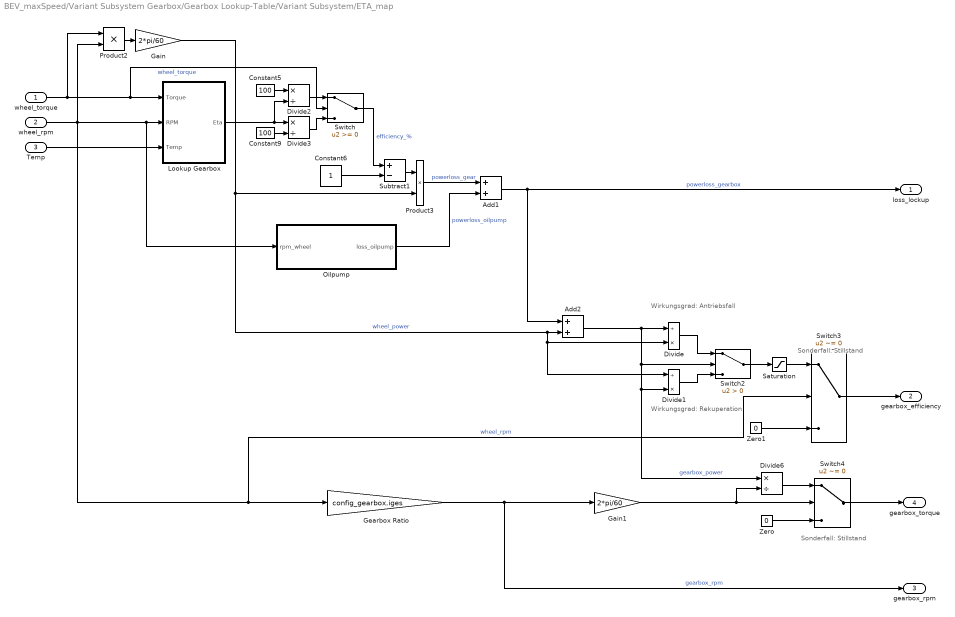
== system BEV_maxSpeed/Variant Subsystem Gearbox/Gearbox Lookup-Table/Variant Subsystem/ETA_map ==
  note: Sonderfall: Stillstand
  note: Sonderfall: Stillstand
  note: Wirkungsgrad:
      | Antriebsfall
  note: Wirkungsgrad:
      | Rekuperation
  wheel_torque : Inport
  wheel_rpm : Inport  Port=2
  Temp : Inport  Port=3
  Add1 : Sum
  Add2 : Sum
  Constant5 : Constant  Value=100
  Constant6 : Constant
  Constant9 : Constant  Value=100
  Divide : Product  Inputs=/*
  Divide1 : Product  Inputs=/*
  Divide2 : Product  Inputs=*/
  Divide3 : Product  Inputs=*/
  Divide6 : Product  Inputs=*/
  Gain : Gain  Gain=2*pi/60
  Gain1 : Gain  Gain=2*pi/60
  Gearbox Ratio : Gain  Gain=config_gearbox.iges
  Lookup Gearbox : Subsystem  Variant=on
  Oilpump : Subsystem
  Product2 : Product  Inputs=**
  Product3 : Product  Inputs=**
  Saturation : Saturate  UpperLimit=inf  LowerLimit=0
  Subtract1 : Sum  Inputs=+-
  Switch : Switch  SaturateOnIntegerOverflow=off  InputSameDT=off
  Switch2 : Switch  Criteria=u2 > Threshold  SaturateOnIntegerOverflow=off  InputSameDT=off
  Switch3 : Switch  Criteria=u2 ~= 0  SaturateOnIntegerOverflow=off  InputSameDT=off
  Switch4 : Switch  Criteria=u2 ~= 0  SaturateOnIntegerOverflow=off  InputSameDT=off
  Zero : Constant  Value=0  OutDataTypeStr=Inherit: Inherit via back propagation
  Zero1 : Constant  Value=0  OutDataTypeStr=Inherit: Inherit via back propagation
  loss_lockup : Outport
  gearbox_efficiency : Outport  Port=2
  gearbox_rpm : Outport  Port=3
  gearbox_torque : Outport  Port=4
  wires:
  wheel_torque/1 -> Lookup Gearbox/1(Torque), Switch/2, Product2/1  "wheel_torque"
  Divide1/1 -> Switch2/3
  Product2/1 -> Gain/1
  wheel_rpm/1 -> Switch3/2, Gearbox Ratio/1, Product2/2, Oilpump/1(rpm_wheel), Lookup Gearbox/2(RPM)  "wheel_rpm"
  Constant6/1 -> Subtract1/2
  Subtract1/1 -> Product3/1
  Switch/1 -> Subtract1/1  "efficiency_%"
  Product3/1 -> Add1/1  "powerloss_gear"
  Zero1/1 -> Switch3/3
  Switch2/1 -> Saturation/1
  Divide2/1 -> Switch/1
  Zero/1 -> Switch4/3
  Switch4/1 -> gearbox_torque/1
  Switch3/1 -> gearbox_efficiency/1
  Divide6/1 -> Switch4/1
  Gearbox Ratio/1 -> Gain1/1, gearbox_rpm/1  "gearbox_rpm"
  Divide3/1 -> Switch/3
  Add2/1 -> Switch2/2, Divide6/1, Divide1/2, Divide/1  "gearbox_power"
  Gain1/1 -> Switch4/2, Divide6/2
  Temp/1 -> Lookup Gearbox/3(Temp)
  Gain/1 -> Product3/2, Divide1/1, Divide/2, Add2/2  "wheel_power"
  Add1/1 -> Add2/1, loss_lockup/1  "powerloss_gearbox"
  Constant9/1 -> Divide3/2
  Oilpump/1(loss_oilpump) -> Add1/2  "powerloss_oilpump"
  Lookup Gearbox/1(Eta) -> Divide2/2, Divide3/1
  Divide/1 -> Switch2/1
  Constant5/1 -> Divide2/1
  Saturation/1 -> Switch3/1

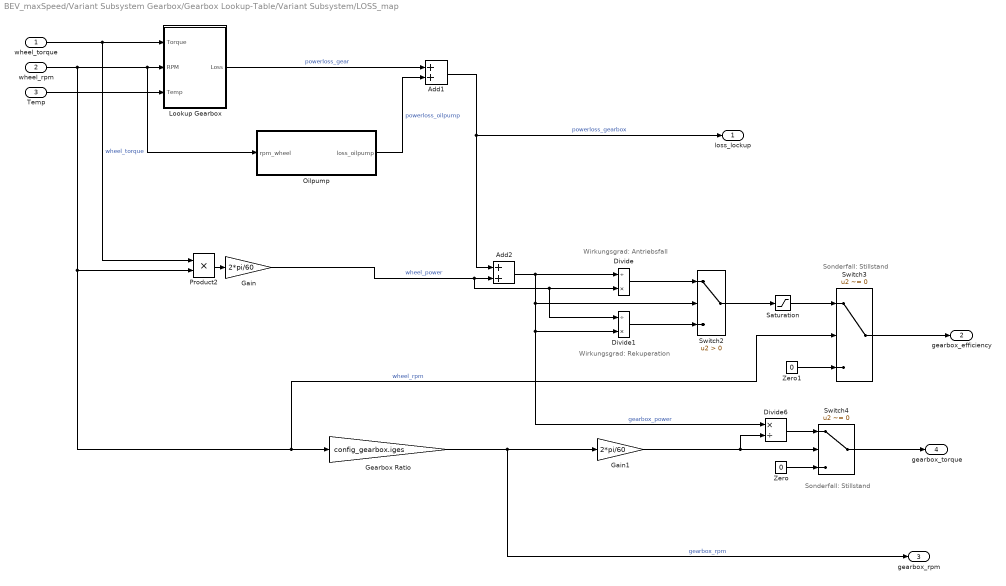
== system BEV_maxSpeed/Variant Subsystem Gearbox/Gearbox Lookup-Table/Variant Subsystem/LOSS_map ==
  note: Sonderfall: Stillstand
  note: Wirkungsgrad: Antriebsfall
  note: Wirkungsgrad: Rekuperation
  note: Sonderfall: Stillstand
  wheel_torque : Inport
  wheel_rpm : Inport  Port=2
  Temp : Inport  Port=3
  Add1 : Sum
  Add2 : Sum
  Divide : Product  Inputs=/*
  Divide1 : Product  Inputs=/*
  Divide6 : Product  Inputs=*/
  Gain : Gain  Gain=2*pi/60
  Gain1 : Gain  Gain=2*pi/60
  Gearbox Ratio : Gain  Gain=config_gearbox.iges
  Lookup Gearbox : Subsystem  Variant=on
  Oilpump : Subsystem
  Product2 : Product  Inputs=**
  Saturation : Saturate  UpperLimit=inf  LowerLimit=0
  Switch2 : Switch  Criteria=u2 > Threshold  SaturateOnIntegerOverflow=off  InputSameDT=off
  Switch3 : Switch  Criteria=u2 ~= 0  SaturateOnIntegerOverflow=off  InputSameDT=off
  Switch4 : Switch  Criteria=u2 ~= 0  SaturateOnIntegerOverflow=off  InputSameDT=off
  Zero : Constant  Value=0  OutDataTypeStr=Inherit: Inherit via back propagation
  Zero1 : Constant  Value=0  OutDataTypeStr=Inherit: Inherit via back propagation
  loss_lockup : Outport
  gearbox_efficiency : Outport  Port=2
  gearbox_rpm : Outport  Port=3
  gearbox_torque : Outport  Port=4
  wires:
  Gain/1 -> Divide1/1, Divide/2, Add2/2  "wheel_power"
  wheel_torque/1 -> Lookup Gearbox/1(Torque), Product2/1  "wheel_torque"
  Lookup Gearbox/1(Loss) -> Add1/1  "powerloss_gear"
  Product2/1 -> Gain/1
  Switch4/1 -> gearbox_torque/1
  Switch3/1 -> gearbox_efficiency/1
  Gearbox Ratio/1 -> gearbox_rpm/1, Gain1/1  "gearbox_rpm"
  Switch2/1 -> Saturation/1
  Divide/1 -> Switch2/1
  Add2/1 -> Divide/1, Switch2/2, Divide1/2, Divide6/1  "gearbox_power"
  Zero/1 -> Switch4/3
  Divide6/1 -> Switch4/1
  Divide1/1 -> Switch2/3
  Oilpump/1(loss_oilpump) -> Add1/2  "powerloss_oilpump"
  Add1/1 -> loss_lockup/1, Add2/1  "powerloss_gearbox"
  Temp/1 -> Lookup Gearbox/3(Temp)
  Gain1/1 -> Switch4/2, Divide6/2
  wheel_rpm/1 -> Switch3/2, Gearbox Ratio/1, Product2/2, Lookup Gearbox/2(RPM), Oilpump/1(rpm_wheel)  "wheel_rpm"
  Zero1/1 -> Switch3/3
  Saturation/1 -> Switch3/1

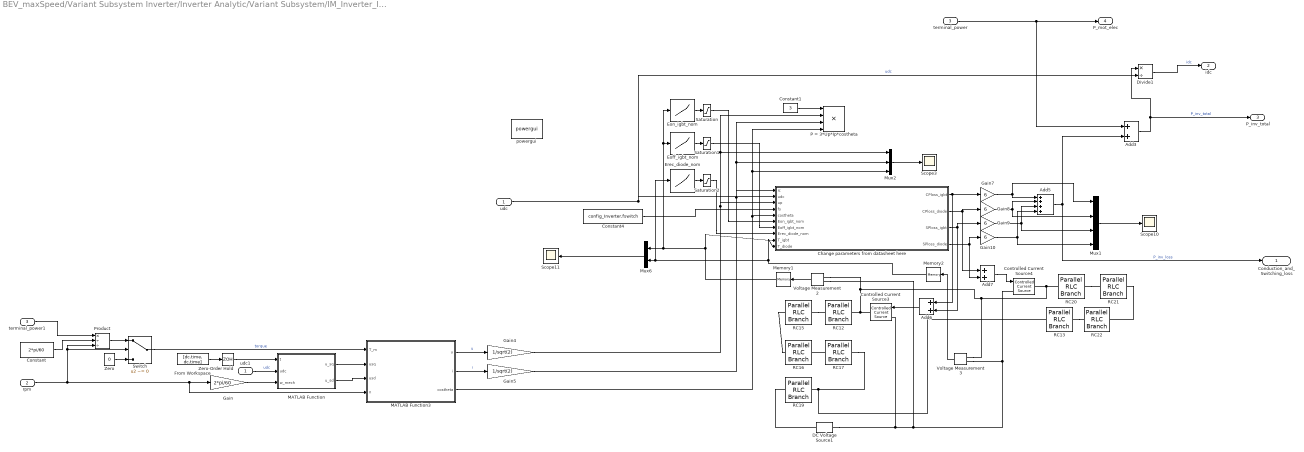
== system BEV_maxSpeed/Variant Subsystem Inverter/Inverter Analytic/Variant Subsystem/IM_Inverter_IGBT_Analytic ==
  udc : Inport
  rpm : Inport  Port=2
  terminal_power : Inport  Port=3
  Add3 : Sum
  Add5 : Sum  Inputs=++++
  Add6 : Sum
  Add7 : Sum
  Change parameters from datasheet here : MATLAB Function  TreatAsAtomicUnit=on
  Constant : Constant  Value=2*pi/60
  Constant1 : Constant  Value=3
  Constant4 : Constant  Value=config_Inverter.fswitch
  Controlled Current Source3 : spsControlledCurrentSourceLib/Controlled Current Source  Initialize=on  Source_Type=AC  Amplitude=0  Phase=0  Frequency=0  Measurements=None
  Controlled Current Source4 : spsControlledCurrentSourceLib/Controlled Current Source  Initialize=on  Source_Type=AC  Amplitude=0  Phase=0  Frequency=0  Measurements=None
  DC Voltage Source1 : spsDCVoltageSourceLib/DC Voltage Source  Amplitude=25  Measurements=None
  Divide1 : Product  Inputs=*/
  Eoff_igbt_nom : Lookup_n-D  NumberOfTableDimensions=1  BreakpointsForDimension1=[25, 150, 175]  Table="[23.5*1e-3,  29*1e-3,  30*1e-3]"  InternalRulePriority=Speed  RndMeth=Simplest
  Eon_igbt_nom : Lookup_n-D  NumberOfTableDimensions=1  BreakpointsForDimension1=[25, 150, 175]  Table="[13.5*1e-3,  17.5*1e-3,  18*1e-3]"  InternalRulePriority=Speed  RndMeth=Simplest
  Erec_diode_nom : Lookup_n-D  NumberOfTableDimensions=1  BreakpointsForDimension1=[25, 150, 175]  Table="[7*1e-3,  13*1e-3,  15*1e-3]"  InternalRulePriority=Speed  RndMeth=Simplest
  From Workspace : FromWorkspace  VariableName=[dc.time, dc.time]
  Gain : Gain  Gain=2*pi/60
  Gain{7..10} (4 alike) : Gain  Gain=6
  Gain4 : Gain  Gain=1/sqrt(2)
  Gain5 : Gain  Gain=1/sqrt(2)
  MATLAB Function : MATLAB Function  TreatAsAtomicUnit=on
  MATLAB Function3 : MATLAB Function  TreatAsAtomicUnit=on
  Memory1 : Memory  InitialCondition=25  InheritSampleTime=on
  Memory2 : Memory  InitialCondition=25  InheritSampleTime=on
  Mux1 : Mux
  Mux2 : Mux  Inputs=3
  Mux6 : Mux  Inputs=2
  P = 3*Up*Ip*costheta : Product  Inputs=4
  Product : Product  Inputs=*//
  RC12 : spsParallelRLCBranchLib/Parallel RLC Branch  LConnTagsString=a  RConnTagsString=__new0  BranchType=RC  Resistance=config_Inverter.R1igbt  Inductance=1e-3  SetiL0=off  InitialCurrent=0  Capacitance=config_Inverter.C1igbt  Setx0=off  InitialVoltage=0  Measurements=None
  RC13 : spsParallelRLCBranchLib/Parallel RLC Branch  LConnTagsString=a  RConnTagsString=__new0  BranchType=RC  Resistance=config_Inverter.R4diode  Inductance=1e-3  SetiL0=off  InitialCurrent=0  Capacitance=config_Inverter.C4diode  Setx0=off  InitialVoltage=0  Measurements=None
  RC15 : spsParallelRLCBranchLib/Parallel RLC Branch  LConnTagsString=a  RConnTagsString=__new0  BranchType=RC  Resistance=config_Inverter.R2igbt  Inductance=1e-3  SetiL0=off  InitialCurrent=0  Capacitance=config_Inverter.C2igbt  Setx0=off  InitialVoltage=0  Measurements=None
  RC16 : spsParallelRLCBranchLib/Parallel RLC Branch  LConnTagsString=a  RConnTagsString=__new0  BranchType=RC  Resistance=config_Inverter.R3igbt  Inductance=1e-3  SetiL0=off  InitialCurrent=0  Capacitance=config_Inverter.C3igbt  Setx0=off  InitialVoltage=0  Measurements=None
  RC17 : spsParallelRLCBranchLib/Parallel RLC Branch  LConnTagsString=a  RConnTagsString=__new0  BranchType=RC  Resistance=config_Inverter.R4igbt  Inductance=1e-3  SetiL0=off  InitialCurrent=0  Capacitance=config_Inverter.C4igbt  Setx0=off  InitialVoltage=0  Measurements=None
  RC19 : spsParallelRLCBranchLib/Parallel RLC Branch  LConnTagsString=a  RConnTagsString=__new0  BranchType=R  Resistance=config_Inverter.R6igbt  Inductance=1e-3  SetiL0=off  InitialCurrent=0  Capacitance=175  Setx0=on  InitialVoltage=0  Measurements=None
  RC20 : spsParallelRLCBranchLib/Parallel RLC Branch  LConnTagsString=a  RConnTagsString=__new0  BranchType=RC  Resistance=config_Inverter.R1diode  Inductance=1e-3  SetiL0=off  InitialCurrent=0  Capacitance=config_Inverter.C1diode  Setx0=off  InitialVoltage=0  Measurements=None
  RC21 : spsParallelRLCBranchLib/Parallel RLC Branch  LConnTagsString=a  RConnTagsString=__new0  BranchType=RC  Resistance=config_Inverter.R2diode  Inductance=1e-3  SetiL0=off  InitialCurrent=0  Capacitance=config_Inverter.C2diode  Setx0=off  InitialVoltage=0  Measurements=None
  RC22 : spsParallelRLCBranchLib/Parallel RLC Branch  LConnTagsString=a  RConnTagsString=__new0  BranchType=RC  Resistance=config_Inverter.R3diode  Inductance=1e-3  SetiL0=off  InitialCurrent=0  Capacitance=config_Inverter.C3diode  Setx0=off  InitialVoltage=0  Measurements=None
  Saturation : Saturate  UpperLimit=18*1e-3  LowerLimit=13.5*1e-3
  Saturation1 : Saturate  UpperLimit=30*1e-3  LowerLimit=23.5*1e-3
  Saturation2 : Saturate  UpperLimit=15*1e-3  LowerLimit=7*1e-3
  Scope10 : Scope
  Scope11 : Scope
  Scope3 : Scope
  Switch : Switch  Criteria=u2 ~= 0  SaturateOnIntegerOverflow=off  InputSameDT=off
  Voltage Measurement2 : spsVoltageMeasurementLib/Voltage Measurement  PhasorSimulation=off  OutputType=Complex  PSBequivalent=0
  Voltage Measurement3 : spsVoltageMeasurementLib/Voltage Measurement  PhasorSimulation=off  OutputType=Complex  PSBequivalent=0
  Zero : Constant  Value=0  OutDataTypeStr=Inherit: Inherit via back propagation
  Zero-Order Hold : ZeroOrderHold  SampleTime=-1
  powergui : spspowerguiLib/powergui  Priority=1  SimulationMode=Discrete  SampleTime=1  frequency=60  Iterations=50  frequencyindice=0  Pbase=100e6  ErrMax=1e-4  UnitsV=kV  UnitsW=MW  buscounter=0  FunctionMessages=on  echomessages=on  EnableUseOfTLC=off  CurrentSourceSwitches=off  DisableSnubberDevices=off  DisableRonSwitches=off  DisableVfSwitches=off  DisplayEquations=off  AutomaticDiscreteSolvers=off  SolverType=Backward Euler  Interpol=off  ExternalGateDelay=off  methode=off  Ts=100  x0status=blocks  SPID=off  SwTol=0  HookPort=off  NonlinearTolerance=1e-4  nMaxIteration=100  ContinueOnMaxIteration=off  RestoreLinks=warning  ResistiveCurrentMeasurement=off  Frange=[0:2:500]  Ylog=off  Xlog=on  ShowGrid=off  save=off  variable=ZData  structure=0  ZoomFFT=off  StartTime=0.0  cycles=1  DisplayStyle=1  fundamental=60  FreqAxis=off  MaxFrequency=1000  frequencyindicesteady=1  RmsSteady=1  display=off
  terminal_power1 : InportShadow  Port=3
  udc1 : InportShadow
  Conduction_and_Switching_loss : Outport
  idc : Outport  Port=2
  P_inv_total : Outport  Port=3
  P_mot_elec : Outport  Port=4
  wires:
  Eon_igbt_nom/1 -> Saturation/1
  Erec_diode_nom/1 -> Saturation2/1
  Eoff_igbt_nom/1 -> Saturation1/1
  Gain4/1 -> Change parameters from datasheet here/3(up), Mux2/1, P = 3*Up*Ip*costheta/2
  Saturation1/1 -> Change parameters from datasheet here/7(Eoff_igbt_nom)
  Switch/1 -> MATLAB Function3/1(T_m)  "torque"
  Divide1/1 -> idc/1  "idc"
  Voltage Measurement3/1 -> Memory2/1
  Change parameters from datasheet here/2(CPloss_diode) -> Add7/1, Gain8/1
  Add7/1 -> Controlled Current Source4/1
  Gain8/1 -> Add5/2, Mux1/2
  Change parameters from datasheet here/3(SPloss_igbt) -> Add6/2, Gain9/1
  Add3/1 -> Divide1/1, P_inv_total/1  "P_inv_total"
  Voltage Measurement2/1 -> Memory1/1
  Mux6/1 -> Scope11/1
  Saturation2/1 -> Change parameters from datasheet here/8(Erec_diode_nom)
  Saturation/1 -> Change parameters from datasheet here/6(Eon_igbt_nom)
  Change parameters from datasheet here/4(SPloss_diode) -> Add7/2, Gain10/1
  Gain9/1 -> Add5/3, Mux1/3
  Mux1/1 -> Scope10/1
  Gain7/1 -> Add5/1, Mux1/1
  Change parameters from datasheet here/1(CPloss_igbt) -> Gain7/1, Add6/1
  Constant4/1 -> Change parameters from datasheet here/4(fs)
  Memory1/1 -> Change parameters from datasheet here/9(T_igbt), Mux6/1, Eoff_igbt_nom/1, Eon_igbt_nom/1
  Memory2/1 -> Mux6/2, Erec_diode_nom/1, Change parameters from datasheet here/10(T_diode)
  Gain10/1 -> Mux1/4, Add5/4
  Constant1/1 -> P = 3*Up*Ip*costheta/1
  Add5/1 -> Add3/2, Conduction_and_Switching_loss/1  "P_inv_loss"
  Add6/1 -> Controlled Current Source3/1
  Mux2/1 -> Scope3/1
  udc/1 -> Divide1/2, Change parameters from datasheet here/2(udc)  "udc"
  MATLAB Function3/3(costheta) -> Mux2/3, P = 3*Up*Ip*costheta/4, Change parameters from datasheet here/5(costheta)
  Gain5/1 -> Change parameters from datasheet here/1(ic), Mux2/2, P = 3*Up*Ip*costheta/3
  MATLAB Function3/1(u) -> Gain4/1  "u"
  MATLAB Function3/2(i) -> Gain5/1  "i"
  MATLAB Function/1(u_sq) -> MATLAB Function3/2(usq)
  MATLAB Function/2(u_sd) -> MATLAB Function3/3(usd)
  Gain/1 -> MATLAB Function/3(w_mech)
  udc1/1 -> MATLAB Function/2(udc)  "udc"
  terminal_power/1 -> Add3/1, P_mot_elec/1
  Zero/1 -> Switch/3
  rpm/1 -> Switch/2, Product/3, MATLAB Function3/4(n), Gain/1
  Constant/1 -> Product/2
  Product/1 -> Switch/1
  terminal_power1/1 -> Product/1
  From Workspace/1 -> Zero-Order Hold/1
  Zero-Order Hold/1 -> MATLAB Function/1(t)
  connections:
  RC15/RConn1 -- RC12/LConn1
  RC17/LConn1 -- RC16/RConn1
  RC15/LConn1 -- RC16/LConn1
  RC20/LConn1 -- RC21/RConn1
  DC Voltage Source1/RConn1 -- RC19/LConn1
  RC13/LConn1 -- RC22/RConn1
  RC21/LConn1 -- RC22/LConn1
  RC17/RConn1 -- RC13/RConn1 -- RC19/RConn1
  Voltage Measurement2/LConn2 -- Voltage Measurement3/LConn2 -- Controlled Current Source4/LConn1 -- DC Voltage Source1/LConn1 -- Controlled Current Source3/LConn1
  RC12/RConn1 -- Controlled Current Source3/RConn1 -- Voltage Measurement2/LConn1 -- Voltage Measurement3/LConn1 -- RC20/RConn1 -- Controlled Current Source4/RConn1

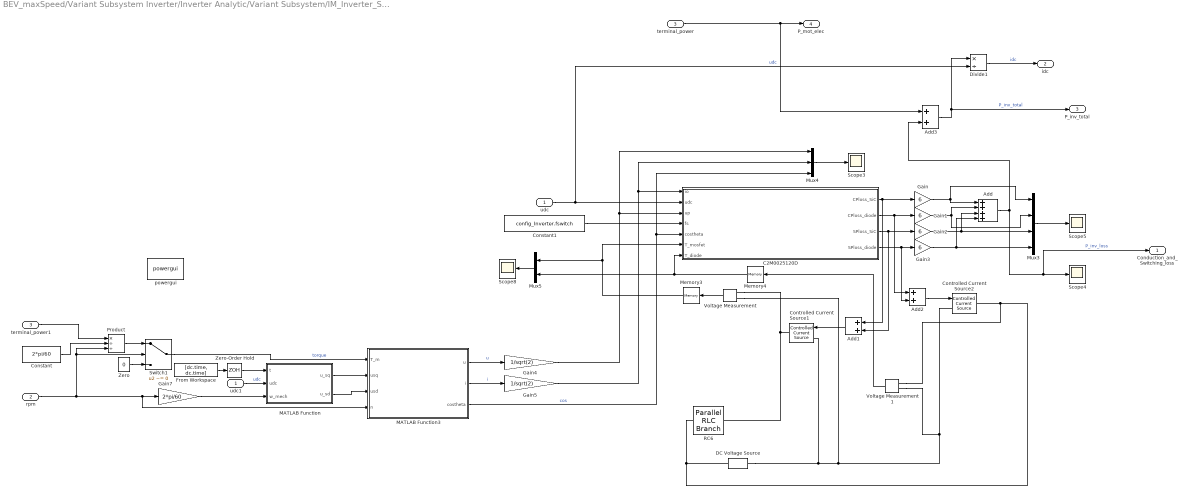
== system BEV_maxSpeed/Variant Subsystem Inverter/Inverter Analytic/Variant Subsystem/IM_Inverter_SiC-MOSFET_Analytic ==
  udc : Inport
  rpm : Inport  Port=2
  terminal_power : Inport  Port=3
  Add : Sum  Inputs=++++
  Add1 : Sum
  Add2 : Sum
  Add3 : Sum
  C2M0025120D : MATLAB Function  TreatAsAtomicUnit=on
  Constant : Constant  Value=2*pi/60
  Constant1 : Constant  Value=config_Inverter.fswitch
  Controlled Current Source1 : spsControlledCurrentSourceLib/Controlled Current Source  Initialize=on  Source_Type=AC  Amplitude=0  Phase=0  Frequency=0  Measurements=None
  Controlled Current Source2 : spsControlledCurrentSourceLib/Controlled Current Source  Initialize=on  Source_Type=AC  Amplitude=0  Phase=0  Frequency=0  Measurements=None
  DC Voltage Source : spsDCVoltageSourceLib/DC Voltage Source  Amplitude=25  Measurements=None
  Divide1 : Product  Inputs=*/
  From Workspace : FromWorkspace  VariableName=[dc.time, dc.time]
  Gain{,1..3} (4 alike) : Gain  Gain=6
  Gain4 : Gain  Gain=1/sqrt(2)
  Gain5 : Gain  Gain=1/sqrt(2)
  Gain7 : Gain  Gain=2*pi/60
  MATLAB Function : MATLAB Function  TreatAsAtomicUnit=on
  MATLAB Function3 : MATLAB Function  TreatAsAtomicUnit=on
  Memory3 : Memory  InitialCondition=25  InheritSampleTime=on
  Memory4 : Memory  InitialCondition=25  InheritSampleTime=on
  Mux3 : Mux
  Mux4 : Mux  Inputs=3
  Mux5 : Mux  Inputs=2
  Product : Product  Inputs=*//
  RC6 : spsParallelRLCBranchLib/Parallel RLC Branch  LConnTagsString=a  RConnTagsString=__new0  BranchType=R  Resistance=config_Inverter.Rmosfet  Inductance=1e-3  SetiL0=off  InitialCurrent=0  Capacitance=175  Setx0=on  InitialVoltage=0  Measurements=None
  Scope{3..5,8} (4 alike) : Scope
  Switch1 : Switch  Criteria=u2 ~= 0  SaturateOnIntegerOverflow=off  InputSameDT=off
  Voltage Measurement : spsVoltageMeasurementLib/Voltage Measurement  PhasorSimulation=off  OutputType=Complex  PSBequivalent=0
  Voltage Measurement1 : spsVoltageMeasurementLib/Voltage Measurement  PhasorSimulation=off  OutputType=Complex  PSBequivalent=0
  Zero : Constant  Value=0  OutDataTypeStr=Inherit: Inherit via back propagation
  Zero-Order Hold : ZeroOrderHold  SampleTime=-1
  powergui : spspowerguiLib/powergui  Priority=1  SimulationMode=Discrete  SampleTime=1  frequency=60  Iterations=50  frequencyindice=0  Pbase=100e6  ErrMax=1e-4  UnitsV=kV  UnitsW=MW  buscounter=0  FunctionMessages=on  echomessages=on  EnableUseOfTLC=off  CurrentSourceSwitches=off  DisableSnubberDevices=off  DisableRonSwitches=off  DisableVfSwitches=off  DisplayEquations=off  AutomaticDiscreteSolvers=off  SolverType=Backward Euler  Interpol=off  ExternalGateDelay=off  methode=off  Ts=100  x0status=blocks  SPID=off  SwTol=0  HookPort=off  NonlinearTolerance=1e-4  nMaxIteration=100  ContinueOnMaxIteration=off  RestoreLinks=warning  ResistiveCurrentMeasurement=off  Frange=[0:2:500]  Ylog=off  Xlog=on  ShowGrid=off  save=off  variable=ZData  structure=0  ZoomFFT=off  StartTime=0.0  cycles=1  DisplayStyle=1  fundamental=60  FreqAxis=off  MaxFrequency=1000  frequencyindicesteady=1  RmsSteady=1  display=off
  terminal_power1 : InportShadow  Port=3
  udc1 : InportShadow
  Conduction_and_Switching_loss : Outport
  idc : Outport  Port=2
  P_inv_total : Outport  Port=3
  P_mot_elec : Outport  Port=4
  wires:
  terminal_power/1 -> Add3/1, P_mot_elec/1
  Add3/1 -> Divide1/1, P_inv_total/1  "P_inv_total"
  Gain5/1 -> Mux4/2, C2M0025120D/1(io)
  Gain4/1 -> Mux4/1, C2M0025120D/3(up)
  udc/1 -> C2M0025120D/2(udc), Divide1/2  "udc"
  Divide1/1 -> idc/1  "idc"
  Add/1 -> Scope4/1, Conduction_and_Switching_loss/1, Add3/2  "P_inv_loss"
  MATLAB Function3/3(costheta) -> Mux4/3, C2M0025120D/5(costheta)  "cos"
  MATLAB Function3/2(i) -> Gain5/1  "i"
  Mux3/1 -> Scope5/1
  Mux4/1 -> Scope3/1
  Voltage Measurement/1 -> Memory3/1
  Mux5/1 -> Scope8/1
  C2M0025120D/2(CPloss_diode) -> Gain1/1, Add2/1
  Constant1/1 -> C2M0025120D/4(fs)
  C2M0025120D/3(SPloss_SiC) -> Gain2/1, Add1/2
  Voltage Measurement1/1 -> Memory4/1
  Add2/1 -> Controlled Current Source2/1
  Memory4/1 -> Mux5/2, C2M0025120D/7(T_diode)
  Add1/1 -> Controlled Current Source1/1
  Gain/1 -> Add/1, Mux3/1
  C2M0025120D/4(SPloss_diode) -> Gain3/1, Add2/2
  Gain1/1 -> Add/2, Mux3/2
  Gain2/1 -> Add/3, Mux3/3
  C2M0025120D/1(CPloss_SiC) -> Gain/1, Add1/1
  Memory3/1 -> C2M0025120D/6(T_mosfet), Mux5/1
  Gain3/1 -> Mux3/4, Add/4
  MATLAB Function/1(u_sq) -> MATLAB Function3/2(usq)
  MATLAB Function/2(u_sd) -> MATLAB Function3/3(usd)
  MATLAB Function3/1(u) -> Gain4/1  "u"
  terminal_power1/1 -> Product/1
  udc1/1 -> MATLAB Function/2(udc)  "udc"
  rpm/1 -> Switch1/2, Product/3, MATLAB Function3/4(n), Gain7/1
  Gain7/1 -> MATLAB Function/3(w_mech)
  Zero/1 -> Switch1/3
  Product/1 -> Switch1/1
  Constant/1 -> Product/2
  Switch1/1 -> MATLAB Function3/1(T_m)  "torque"
  From Workspace/1 -> Zero-Order Hold/1
  Zero-Order Hold/1 -> MATLAB Function/1(t)
  connections:
  RC6/RConn1 -- Controlled Current Source1/RConn1 -- Voltage Measurement/LConn1
  Controlled Current Source2/LConn1 -- Voltage Measurement/LConn2 -- Controlled Current Source1/LConn1 -- DC Voltage Source/LConn1 -- Voltage Measurement1/LConn2
  Voltage Measurement1/LConn1 -- Controlled Current Source2/RConn1 -- RC6/LConn1 -- DC Voltage Source/RConn1
